simulink model "debugECDD"  (Simulink 7.2)
settings: Solver=ode1  StartTime=0.0  StopTime=50  FixedStep=0.002  RelTol=1e-3
values from neighbouring files (symbols this model uses):
  a = param.a    [DSC_Control_Analysis.m]    (also in DSC_Control_Analysis_Exp.m; DSC_Speed_Control_Analysis.m; EmpiricalTireCurves.m = 1.35; FFW_Fx.m = sqrt(curvature/(2*clothoidLength)))
  b = 1.15    [EmpiricalTireCurves.m]
  Cfls = Cfl    [EC_params_nissan.m]
  Crls = Crl    [EC_params_nissan.m]
  Iz = param.Iz    [DSC_Control_Analysis.m]    (also in DSC_Control_Analysis_Exp.m; DSC_Speed_Control_Analysis.m; EmpiricalTireCurves.m = 1300)
  K = 10    [EC_params_nissan.m]
  Ks = -10    [EC_params_nissan.m]
  Ksl = -10    [EC_params_nissan.m]
  Kt = 40000    [EC_params_nissan.m]
  Ku = -40000    [EC_params_nissan.m]
  m = 1724    [EmpiricalTireCurves.m]
  mu_s = mu_p    (= 0.6)    [EC_params_nissan.m]    (also in EmpiricalTireCurves.m = 0.55)
  Ns = 10    [EC_params_nissan.m]
  q = 1    [EC_params_nissan.m]
undefined symbols (not defined in the file or in its folder): c, Cfl, Crl, dden, denafilt, dnum, filtera, filterb, h_roll, Ifalphaparam, numafilt, param, rfl, rfr, rrl, rrr, sglu, slimFxl, slimFxu, sliml, slimMll, slimMlr, slimMul, slimMur, slimu, steering_limit, tw_m, wc
libraries: simulink x15, xpclib x3, UserBlocks x1
(part 1 of 3)
settings Model: Creator=joe4016  LastModifiedBy=joe4016
settings DataIOCC: LimitDataPoints=off

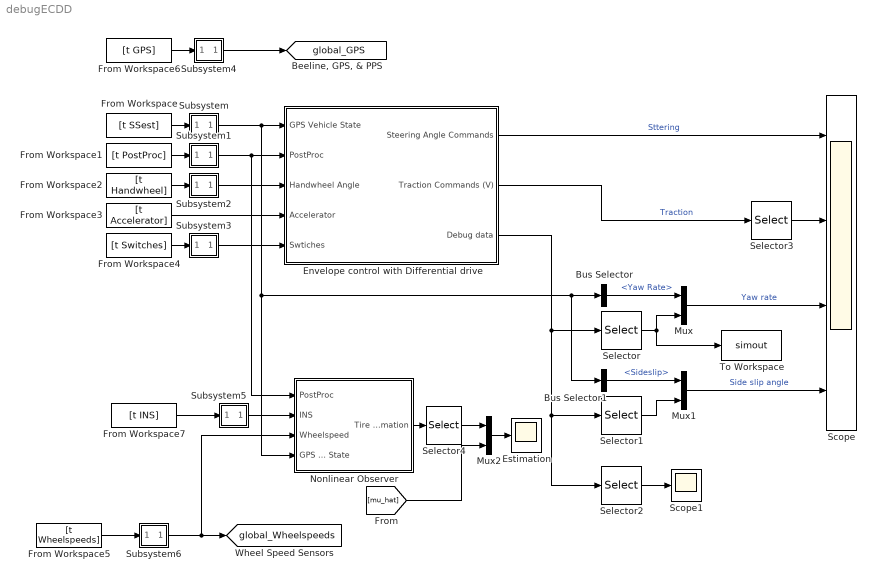
== system debugECDD ==
  Bus Selector : BusSelector  OutputSignals=Yaw Rate
  Bus Selector1 : BusSelector  OutputSignals=Sideslip
  Envelope control with Differential drive : Subsystem  AncestorBlock=UserBlocks/Envelope control with Differential drive
      mask init:
      | % get P1 parameters
      | p1_params;
      | 
      | % get params to filter handwheel angle
      | SteeringController;
      | 
      | Ts=0.002;
  Estimation : Scope
      settings: SaveName=ScopeData9
  From Workspace : FromWorkspace  VariableName=[t SSest]  SampleTime=0.002
  From Workspace1 : FromWorkspace  VariableName=[t PostProc]  SampleTime=0.002
  From Workspace2 : FromWorkspace  VariableName=[t Handwheel]  SampleTime=0.002
  From Workspace3 : FromWorkspace  VariableName=[t Accelerator]  SampleTime=0.002
  From Workspace4 : FromWorkspace  VariableName=[t Switches]  SampleTime=0.002
  From Workspace5 : FromWorkspace  VariableName=[t Wheelspeeds]  SampleTime=0.002
  From Workspace6 : FromWorkspace  VariableName=[t GPS]  SampleTime=0.002
  From Workspace7 : FromWorkspace  VariableName=[t INS]  SampleTime=0.002
  Mux : Mux  Inputs=2
  Mux1 : Mux  Inputs=2
  Mux2 : Mux  Inputs=2
  Nonlinear Observer : Subsystem
      mask init:
      | p1_params
      | nissan_steer_lookup_data
      | If_alpha_params
      | [filterb,filtera]=butter(5,0.02);
      | Ts=0.002;
      | 
      | % dryasphalt = 1;
      | % gravel = 2;
      | % 
      | % AtShoreline = [gcs '/Nonlinear Observer' '/Enable Shoreline Gravel'];
      | % 
      | % % default is dryasphalt
      | % set_param(AtShoreline, 'value', '0');
      | % 
      | % % if gravel selected, make constant AtShoreline = 1
      | % if (roadsurface == gravel)
      | %     set_param(AtShoreline, 'value', '1');
      | % end
      | %
  Scope : Scope  NumInputPorts=4
      settings: TimeRange=120  YMin=-0.4~0.5~-1.334911242603574~-0.5153846153846171  YMax=0.6~3~1.597633136094648~0.638461538461538
  Scope1 : Scope
  Selector : Selector  InputPortWidth=32  IndexOptions=Index vector (dialog)  Indices=[25 20 21]  OutputSizes=1
  Selector1 : Selector  InputPortWidth=32  IndexOptions=Index vector (dialog)  Indices=[24 22 23]  OutputSizes=1
  Selector2 : Selector  InputPortWidth=32  IndexOptions=Index vector (dialog)  Indices=16  OutputSizes=1
  Selector3 : Selector  InputPortWidth=2  IndexOptions=Index vector (dialog)  Indices=[2 1]  OutputSizes=1
  Selector4 : Selector  InputPortWidth=3  IndexOptions=Index vector (dialog)  Indices=2  OutputSizes=1
  Subsystem : Subsystem
  Subsystem1 : Subsystem
  Subsystem2 : Subsystem
  Subsystem3 : Subsystem
  Subsystem4 : Subsystem
  Subsystem5 : Subsystem
  Subsystem6 : Subsystem
  To Workspace : ToWorkspace  VariableName=simout  SampleTime=-1  SaveFormat=Array
  tag scope: global_GPS=global, global_Wheelspeeds=global
  wires:
  From Workspace/1 -> Subsystem/1(In1)
  From Workspace1/1 -> Subsystem1/1(In1)
  From Workspace2/1 -> Subsystem2/1(In1)
  From Workspace3/1 -> Envelope control with Differential drive/4(Accelerator)
  From Workspace4/1 -> Subsystem3/1(In1)
  Subsystem/1(Out1) -> Envelope control with Differential drive/1(GPS Vehicle State), Bus Selector/1, Bus Selector1/1, Nonlinear Observer/4(GPS Vehicle State)
  Subsystem1/1(Out1) -> Envelope control with Differential drive/2(PostProc), Nonlinear Observer/1(PostProc)
  Subsystem2/1(Out1) -> Envelope control with Differential drive/3(Handwheel Angle)
  Subsystem3/1(Out1) -> Envelope control with Differential drive/5(Swtiches)
  From Workspace5/1 -> Subsystem6/1(In1)
  From Workspace6/1 -> Subsystem4/1(In1)
  Subsystem4/1(Out1) -> [global_GPS]
  Envelope control with Differential drive/1(Steering Angle Commands) -> Scope/1  "Sttering"
  Envelope control with Differential drive/2(Traction Commands (V)) -> Selector3/1  "Traction"
  Envelope control with Differential drive/3(Debug data) -> Selector/1, Selector1/1, Selector2/1
  Mux/1 -> Scope/3  "Yaw rate"
  Selector/1 -> Mux/2, To Workspace/1
  Bus Selector/1 -> Mux/1  "<Yaw Rate>"
  Selector1/1 -> Mux1/2
  Bus Selector1/1 -> Mux1/1  "<Sideslip>"
  Mux1/1 -> Scope/4  "Side slip angle"
  Selector2/1 -> Scope1/1
  Selector3/1 -> Scope/2
  Subsystem5/1(Out1) -> Nonlinear Observer/2(INS)
  From Workspace7/1 -> Subsystem5/1(In1)
  Subsystem6/1(Out1) -> [global_Wheelspeeds], Nonlinear Observer/3(Wheelspeed)
  Nonlinear Observer/1(Tire Estimation) -> Selector4/1
  Mux2/1 -> Estimation/1
  [mu_hat] -> Mux2/2
  Selector4/1 -> Mux2/1

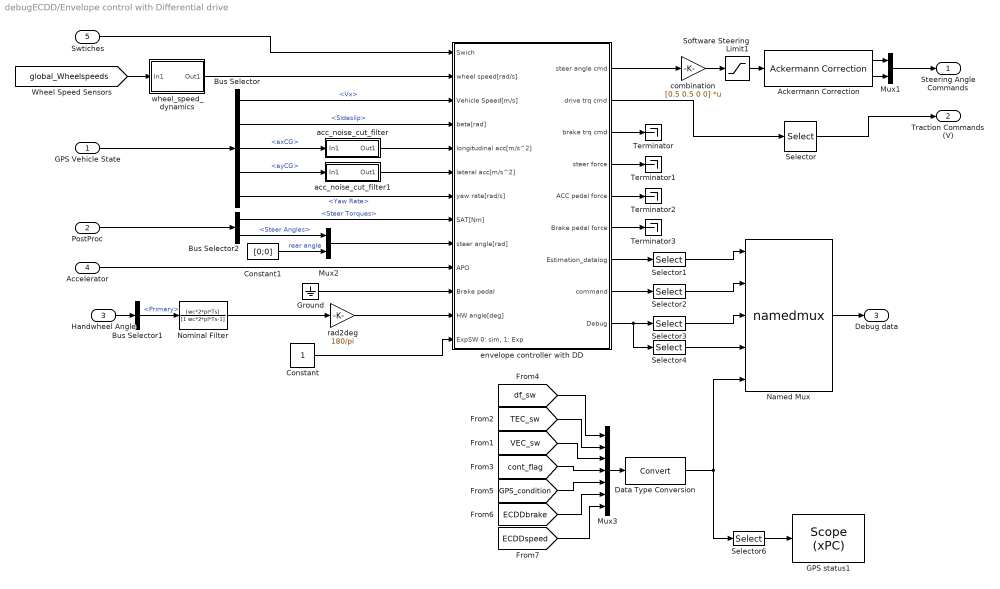
== system debugECDD/Envelope control with Differential drive ==
  GPS Vehicle State : Inport  OutDataType=sfix(16)  OutScaling=2^0
  PostProc : Inport  Port=2  OutDataType=sfix(16)  OutScaling=2^0
  Handwheel Angle : Inport  Port=3  OutDataType=sfix(16)  OutScaling=2^0
  Accelerator : Inport  Port=4  OutDataType=sfix(16)  OutScaling=2^0
  Swtiches : Inport  Port=5  OutDataType=sfix(16)  OutScaling=2^0
  Ackermann Correction : UserBlocks/Steering Controller/Ackermann Correction  SystemSampleTime=-1
  Bus Selector : BusSelector  OutputSignals=Vx,Sideslip,axCG,ayCG,Yaw Rate
  Bus Selector1 : BusSelector  OutputSignals=Primary
  Bus Selector2 : BusSelector  OutputSignals=Steer Torques,Steer Angles
  Constant : Constant  OutDataType=sfix(16)  OutScaling=2^0
  Constant1 : Constant  Value=[0;0]  OutDataType=sfix(16)  OutScaling=2^0
  Data Type Conversion : DataTypeConversion  OutDataType=sfix(16)  OutScaling=2^0
  GPS status1 : xpclib/Misc./Scope (xPC)   SystemSampleTime=-1  scopeno=2  scopetype=Target  autostart=on  viewmode=Numerical  formatstr='%15.6f'  grid=on  ylimits=[-10,10]  nosamples=round(1/Ts)  noprepostsamples=0  interleave=1  triggermode=FreeRun  triggersignal=1  triggerlevel=0.0  triggerslope=Either  triggerscope=1  triggersample=0  filename=data.dat  mode=Lazy  writesize=512  autorestart=off
  Ground : Ground
  Mux1 : Mux  Inputs=2
  Mux2 : Mux  Inputs=2
  Mux3 : Mux  Inputs=7
  Named Mux : S-Function  FunctionName=namedmux  Parameters=inputcount,inputsizes  EnableBusSupport=off  mask{fname=datadescTCS}
      mask prompts: fname "Data description function name"
      mask help:
      | Combines input signals into a single output vector, according to a structure that provides the names and sizes of each signal.
      |
      | The parameter below should be set to the name of a function which returns a 1xN structure array, where N is the number of input signals.  The structure should contain fields "size" which specifies the width of the input signal, and "name" which specifies its name.
      mask init:
      | desc=eval(fname);
      | %if(class(desc)~='cell')
      | %	error('Incorrect description');
      | %end
      | inputcount=length(desc);
      | if((inputcount<1)|(inputcount>50))
      | 	error('Inappropriate number of inputs.');
      | end
      | 
      | inputsizes=[desc.size];
      | 
      | x=min(inputcount*ones(1,50),1:50);
      mask Display:
      | port_label('input',x(1),desc(x(1)).name);
      | port_label('input',x(2),desc(x(2)).name);
      | port_label('input',x(3),desc(x(3)).name);
      | port_label('input',x(4),desc(x(4)).name);
      | port_label('input',x(5),desc(x(5)).name);
      | port_label('input',x(6),desc(x(6)).name);
      | port_label('input',x(7),desc(x(7)).name);
      | port_label('input',x(8),desc(x(8)).name);
      | port_label('input',x(9),desc(x(9)).name);
      | port_label('input',x(10),desc(x(10)).name);
      | port_label('input',x(11),desc(x(11)).name);
      | port_label('input',x(12),desc(x(12)).name);
      | port_label('input',x(13),desc(x(13)).name);
      | port_label('input',x(14),desc(x(14)).name);
      | port_label('input',x(15),desc(x(15)).name);
      | port_label('input',x(16),desc(x(16)).name);
      | port_label('input',x(17),desc(x(17)).name);
      | port_label('input',x(18),desc(x(18)).name);
      | port_label('input',x(19),desc(x(19)).name);
      | port_label('input',x(20),desc(x(20)).name);
      | port_label('input',x(21),desc(x(21)).name);
      | port_label('input',x(22),desc(x(22)).name);
      | port_label('input',x(23),desc(x(23)).name);
      | port_label('input',x(24),desc(x(24)).name);
      | port_label('input',x(25),desc(x(25)).name);
      | port_label('input',x(26),desc(x(26)).name);
      | port_label('input',x(27),desc(x(27)).name);
      | port_label('input',x(28),desc(x(28)).name);
      | port_label('input',x(29),desc(x(29)).name);
      | port_label('input',x(30),desc(x(30)).name);
  Nominal Filter : DiscreteFilter  Numerator=[wc*2*pi*Ts]  Denominator=[1 wc*2*pi*Ts-1]  SampleTime=Ts
  Selector : Selector  InputPortWidth=4  IndexOptions=Index vector (dialog)  Indices=[4 3]  OutputSizes=1
  Selector1 : Selector  InputPortWidth=17  IndexOptions=Index vector (dialog)  Indices=[1:4]  OutputSizes=1
  Selector2 : Selector  InputPortWidth=9  IndexOptions=Index vector (dialog)  Indices=[7:9]  OutputSizes=1
  Selector3 : Selector  InputPortWidth=19  IndexOptions=Index vector (dialog)  Indices=[1:8]  OutputSizes=1
  Selector4 : Selector  InputPortWidth=19  IndexOptions=Index vector (dialog)  Indices=[9,11:19]  OutputSizes=1
  Selector6 : Selector  InputPortWidth=7  IndexOptions=Index vector (dialog)  Indices=[4:7]  OutputSizes=1
  Software Steering Limit1 : Saturate  UpperLimit=steering_limit*pi/180  LowerLimit=-steering_limit*pi/180
  Terminator{,1..3} (4 alike) : Terminator
  acc_noise_cut_filter : Subsystem
      mask init:
      | [numafilt,denafilt]=butter(2,0.02);
  acc_noise_cut_filter1 : Subsystem
      mask init:
      | [numafilt,denafilt]=butter(2,0.02);
  combination : Gain  Gain=[0.5 0.5 0 0]  Multiplication=Matrix(K*u)  ParameterDataType=sfix(16)  ParameterScaling=2^0  OutDataType=sfix(16)  OutScaling=2^0
  envelope controller with DD : Subsystem
      mask init:
      | p1_params
  rad2deg : Gain  Gain=180/pi  ParameterDataType=sfix(16)  ParameterScaling=2^0  OutDataType=sfix(16)  OutScaling=2^0
  wheel_speed_dynamics : Subsystem
      mask init:
      | p1_params
      | EC_params_nissan
      | [filterb,filtera]=butter(2,0.03);
  Steering Angle Commands : Outport  OutDataType=sfix(16)  OutScaling=2^0
  Traction Commands (V) : Outport  Port=2  OutDataType=sfix(16)  OutScaling=2^0
  Debug data : Outport  Port=3  OutDataType=sfix(16)  OutScaling=2^0
  wires:
  Mux3/1 -> Data Type Conversion/1
  Swtiches/1 -> envelope controller with DD/1(Swich)
  envelope controller with DD/1(steer angle cmd) -> combination/1
  [global_Wheelspeeds] -> wheel_speed_dynamics/1(In1)
  wheel_speed_dynamics/1(Out1) -> envelope controller with DD/2(wheel speed[rad/s])
  Bus Selector/4 -> acc_noise_cut_filter1/1(In1)  "<ayCG>"
  Bus Selector/3 -> acc_noise_cut_filter/1(In1)  "<axCG>"
  Bus Selector/2 -> envelope controller with DD/4(beta[rad])  "<Sideslip>"
  Bus Selector/5 -> envelope controller with DD/7(yaw rate[rad/s])  "<Yaw Rate>"
  Bus Selector/1 -> envelope controller with DD/3(Vehicle Speed[m/s])  "<Vx>"
  Accelerator/1 -> envelope controller with DD/10(APO)
  Constant1/1 -> Mux2/2  "rear angle"
  Bus Selector2/2 -> Mux2/1  "<Steer Angles>"
  Bus Selector2/1 -> envelope controller with DD/8(SAT[Nm])  "<Steer Torques>"
  PostProc/1 -> Bus Selector2/1
  GPS Vehicle State/1 -> Bus Selector/1
  Constant/1 -> envelope controller with DD/13("ExpSW 0: sim, 1: Exp")
  rad2deg/1 -> envelope controller with DD/12(HW angle[deg])
  Nominal Filter/1 -> rad2deg/1
  Bus Selector1/1 -> Nominal Filter/1  "<Primary>"
  Named Mux/1 -> Debug data/1
  Selector3/1 -> Named Mux/3
  Selector2/1 -> Named Mux/2
  Selector1/1 -> Named Mux/1
  envelope controller with DD/9(Debug) -> Selector4/1, Selector3/1
  envelope controller with DD/8(command) -> Selector2/1
  envelope controller with DD/2(drive trq cmd) -> Selector/1
  envelope controller with DD/7(Estimation_datalog) -> Selector1/1
  envelope controller with DD/6(Brake pedal force) -> Terminator3/1
  envelope controller with DD/5(ACC pedal force) -> Terminator2/1
  envelope controller with DD/4(steer force) -> Terminator1/1
  envelope controller with DD/3(brake trq cmd) -> Terminator/1
  Selector/1 -> Traction Commands (V)/1
  combination/1 -> Software Steering Limit1/1
  Mux1/1 -> Steering Angle Commands/1
  Ackermann Correction/2 -> Mux1/2
  Ackermann Correction/1 -> Mux1/1
  Software Steering Limit1/1 -> Ackermann Correction/1
  Mux2/1 -> envelope controller with DD/9(steer angle[rad])
  Ground/1 -> envelope controller with DD/11(Brake pedal)
  Handwheel Angle/1 -> Bus Selector1/1
  Data Type Conversion/1 -> Selector6/1, Named Mux/5
  acc_noise_cut_filter/1(Out1) -> envelope controller with DD/5(longitudinal acc[m/s^2])
  acc_noise_cut_filter1/1(Out1) -> envelope controller with DD/6(lateral acc[m/s^2])
  Selector4/1 -> Named Mux/4
  [df_sw] -> Mux3/1
  [TEC_sw] -> Mux3/2
  [VEC_sw] -> Mux3/3
  [cont_flag] -> Mux3/4
  [GPS_condition] -> Mux3/5
  [ECDDbrake] -> Mux3/6
  [ECDDspeed] -> Mux3/7
  Selector6/1 -> GPS status1/1

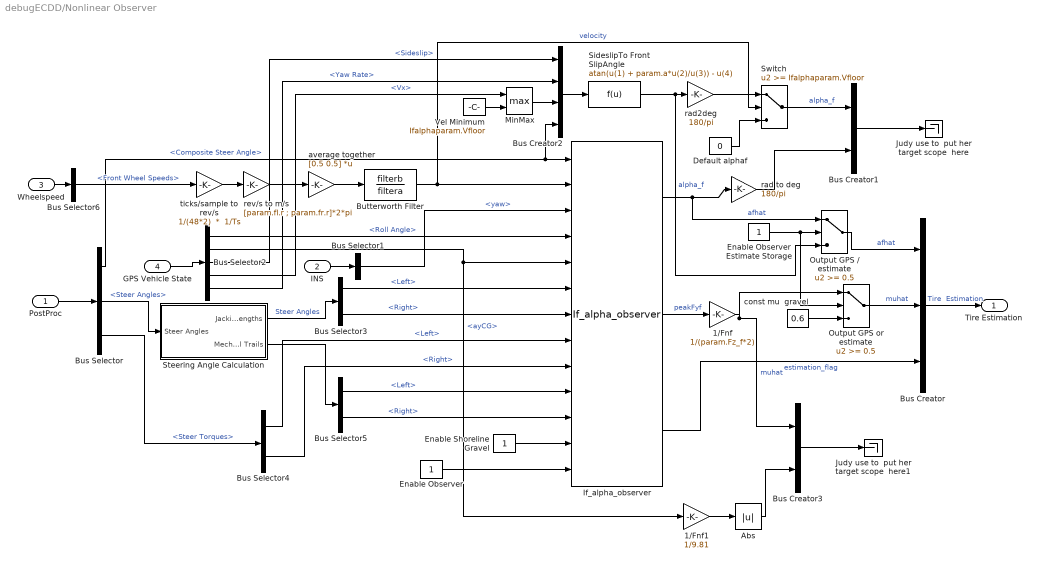
== system debugECDD/Nonlinear Observer ==
  PostProc : Inport  OutDataType=sfix(16)  OutScaling=2^0
  INS : Inport  Port=2  OutDataType=sfix(16)  OutScaling=2^0
  Wheelspeed : Inport  Port=3  OutDataType=sfix(16)  OutScaling=2^0
  GPS Vehicle State : Inport  Port=4  OutDataType=sfix(16)  OutScaling=2^0
  1/Fnf : Gain  Gain=1/(param.Fz_f*2)  ParameterDataType=sfix(16)  ParameterScaling=2^0  OutDataType=sfix(16)  OutScaling=2^0
  1/Fnf1 : Gain  Gain=1/9.81  ParameterDataType=sfix(16)  ParameterScaling=2^0  OutDataType=sfix(16)  OutScaling=2^0
  Abs : Abs
  Bus Creator : BusCreator  Inputs=3
  Bus Creator1 : BusCreator  Inputs=2
  Bus Creator2 : BusCreator
  Bus Creator3 : BusCreator  Inputs=2
  Bus Selector : BusSelector  OutputSignals=Composite Steer Angle,Steer Angles,Steer Torques
  Bus Selector1 : BusSelector  OutputSignals=yaw
  Bus Selector2 : BusSelector  OutputSignals=Roll Angle,ayCG,Sideslip,Vx,Yaw Rate
  Bus Selector3 : BusSelector  OutputSignals=Left,Right
  Bus Selector4 : BusSelector  OutputSignals=Left,Right
  Bus Selector5 : BusSelector  OutputSignals=Left,Right
  Bus Selector6 : BusSelector  OutputSignals=Front Wheel Speeds
  Butterworth Filter : DiscreteFilter  Numerator=filterb  Denominator=filtera  SampleTime=Ts
  Default alphaf : Constant  Value=0  OutDataType=sfix(16)  OutScaling=2^0
  Enable Observer : Constant  OutDataType=sfix(16)  OutScaling=2^0
  Enable Shoreline Gravel : Constant  OutDataType=sfix(16)  OutScaling=2^0
  Enable Observer Estimate Storage : Constant  OutDataType=sfix(16)  OutScaling=2^0
  If_alpha_observer : S-Function  FunctionName=If_alpha_observer  Parameters=|  EnableBusSupport=off
      | Ifalphaparam.tp_window, Ifalphaparam.FIRwindow, Ifalphaparam.IFwindow, param.Fz_f, Ifalphaparam.mu_peak_nom, param.fl.fw, param.fl.Jw, param.fl.bw,
      | 
      | 
      | 
      | 
      | 
      | 
      | 
      | 
      | param.fr.fw, param.fr.Jw, param.fr.bw, param.a, param.b, param.m, Ifalphaparam.hf, param.tw, param.Iz, Ifalphaparam.Kaf0, Ts, Ifalphaparam.phiceil,
      | 
      | 
      | 
      | 
      | 
      | 
      | 
      | 
      | Ifalphaparam.Vfloor, Ifalphaparam.ayfloor, Ifalphaparam.tp0, Ifalphaparam.Caf, Ifalphaparam.Car, Ifalphaparam.Caf_shoreline_sf, Ifalphaparam.mu_slip_nom, 
      | 
      | 
      | 
      | 
      | 
      | 
      | 
      | 
      | Ifalphaparam.alpha_thres, Ifalphaparam.tpthres_sf, Ifalphaparam.Kphif, Ifalphaparam.afhatceil, Ifalphaparam.Kaf_sf_Shoreline, Ifalphaparam.Kaf_sf_asphalt,
      | 
      | 
      | 
      | 
      | 
      | 
      | 
      | 
      | Ifalphaparam.Car_shoreline_sf, Ifalphaparam.alphafoffset, Ifalphaparam.alpharoffset
  Judy use to  put her target scope  here : Terminator
  Judy use to  put her target scope  here1 : Terminator
  MinMax : MinMax  Function=max  Inputs=2  OutDataType=sfix(16)  OutScaling=2^0
  Output GPS / estimate : Switch  Threshold=0.5
  Output GPS or estimate : Switch  Threshold=0.5
  SideslipTo Front SlipAngle : Fcn  Expr=atan(u(1) + param.a*u(2)/u(3)) - u(4)
  Steering Angle Calculation : Subsystem
      mask init:
      | p1_params
      | nissan_steer_lookup_data
  Switch : Switch  Threshold=Ifalphaparam.Vfloor
  Vel Minimum : Constant  Value=Ifalphaparam.Vfloor  OutDataType=sfix(16)  OutScaling=2^0
  average together : Gain  Gain=[0.5 0.5]  Multiplication=Matrix(K*u)  ParameterDataType=sfix(16)  ParameterScaling=2^0  OutDataType=sfix(16)  OutScaling=2^0
  const mu  gravel : Constant  Value=0.6  OutDataType=sfix(16)  OutScaling=2^0
  rad to deg : Gain  Gain=180/pi  ParameterDataType=sfix(16)  ParameterScaling=2^0  OutDataType=sfix(16)  OutScaling=2^0
  rad2deg : Gain  Gain=180/pi  ParameterDataType=sfix(16)  ParameterScaling=2^0  OutDataType=sfix(16)  OutScaling=2^0
  rev/s to m/s : Gain  Gain=[param.fl.r ; param.fr.r]*2*pi  ParameterDataType=sfix(16)  ParameterScaling=2^0  OutDataType=sfix(16)  OutScaling=2^0
  ticks/sample to rev/s : Gain  Gain="1/(48*2)  *  1/Ts"  ParameterDataType=sfix(16)  ParameterScaling=2^0  OutDataType=sfix(16)  OutScaling=2^0
  Tire Estimation : Outport  OutDataType=sfix(16)  OutScaling=2^0
  wires:
  PostProc/1 -> Bus Selector/1
  Bus Creator/1 -> Tire Estimation/1  "Tire  Estimation"
  INS/1 -> Bus Selector1/1
  GPS Vehicle State/1 -> Bus Selector2/1
  Wheelspeed/1 -> Bus Selector6/1
  ticks/sample to rev/s/1 -> rev/s to m/s/1
  rev/s to m/s/1 -> average together/1
  average together/1 -> Butterworth Filter/1
  Bus Selector/2 -> Steering Angle Calculation/1(Steer Angles)  "<Steer Angles>"
  Bus Selector/1 -> If_alpha_observer/1, Bus Creator2/4  "<Composite Steer Angle>"
  Butterworth Filter/1 -> If_alpha_observer/2, Switch/2  "velocity"
  Bus Selector1/1 -> If_alpha_observer/3  "<yaw>"
  Bus Selector2/1 -> If_alpha_observer/4  "<Roll Angle>"
  Bus Selector2/2 -> If_alpha_observer/5, 1/Fnf1/1  "<ayCG>"
  Steering Angle Calculation/1(Jacking Arm Lengths) -> Bus Selector3/1  "Steer Angles"
  Bus Selector3/1 -> If_alpha_observer/6  "<Left>"
  Bus Selector3/2 -> If_alpha_observer/7  "<Right>"
  Bus Selector/3 -> Bus Selector4/1  "<Steer Torques>"
  Bus Selector4/1 -> If_alpha_observer/8  "<Left>"
  Bus Selector4/2 -> If_alpha_observer/9  "<Right>"
  Steering Angle Calculation/2(Mechanical Trails) -> Bus Selector5/1
  Bus Selector5/1 -> If_alpha_observer/10  "<Left>"
  Bus Selector5/2 -> If_alpha_observer/11  "<Right>"
  If_alpha_observer/1 -> rad to deg/1, Output GPS / estimate/1  "afhat"
  If_alpha_observer/3 -> Bus Creator/3  "estimation_flag"
  Bus Selector2/3 -> Bus Creator2/1  "<Sideslip>"
  Bus Creator2/1 -> SideslipTo Front SlipAngle/1
  SideslipTo Front SlipAngle/1 -> rad2deg/1, Output GPS / estimate/3  "alpha_f"
  If_alpha_observer/2 -> 1/Fnf/1  "peakFyf"
  Enable Shoreline Gravel/1 -> If_alpha_observer/12
  1/Fnf1/1 -> Abs/1
  Bus Creator3/1 -> Judy use to  put her target scope  here1/1
  Abs/1 -> Bus Creator3/2
  rad to deg/1 -> Bus Creator1/2
  Bus Creator1/1 -> Judy use to  put her target scope  here/1
  MinMax/1 -> Bus Creator2/3
  Vel Minimum/1 -> MinMax/2
  rad2deg/1 -> Switch/1
  Switch/1 -> Bus Creator1/1  "alpha_f"
  1/Fnf/1 -> Bus Creator3/1, Output GPS or estimate/1  "muhat"
  Default alphaf/1 -> Switch/3
  Enable Observer Estimate Storage/1 -> Output GPS / estimate/2, Output GPS or estimate/2
  Output GPS / estimate/1 -> Bus Creator/1  "afhat"
  Output GPS or estimate/1 -> Bus Creator/2  "muhat"
  const mu  gravel/1 -> Output GPS or estimate/3
  Bus Selector2/4 -> MinMax/1  "<Vx>"
  Bus Selector2/5 -> Bus Creator2/2  "<Yaw Rate>"
  Enable Observer/1 -> If_alpha_observer/13
  Bus Selector6/1 -> ticks/sample to rev/s/1  "<Front Wheel Speeds>"

== system debugECDD/Subsystem ==
  In1 : Inport  OutDataType=sfix(16)  OutScaling=2^0
  Demux : Demux  Outputs=21
  Mux : Mux  Inputs=21
  Out1 : Outport  OutDataType=sfix(16)  OutScaling=2^0
  wires:
  In1/1 -> Demux/1
  Mux/1 -> Out1/1
  Demux/1 -> Mux/1  "Yaw Angle"
  Demux/2 -> Mux/2  "Yaw Gyro Sf"
  Demux/3 -> Mux/3  "Yaw Gyro Bias"
  Demux/4 -> Mux/4  "Yaw Rate"
  Demux/5 -> Mux/5  "Roll Angle"
  Demux/6 -> Mux/6  "Roll Gyro Sf"
  Demux/7 -> Mux/7  "Roll Gyro Bias"
  Demux/8 -> Mux/8  "Roll Rate"
  Demux/9 -> Mux/9  "Vx"
  Demux/10 -> Mux/10  "ax bias"
  Demux/11 -> Mux/11  "axCG"
  Demux/12 -> Mux/12  "VyCG"
  Demux/13 -> Mux/13  "ay bias"
  Demux/14 -> Mux/14  "ayCG"
  Demux/15 -> Mux/15  "Sideslip"
  Demux/16 -> Mux/16  "Pos E"
  Demux/17 -> Mux/17  "Pos N"
  Demux/18 -> Mux/18  "OEM4 Delay"
  Demux/19 -> Mux/19  "Beeline Delay"
  Demux/20 -> Mux/20  "OEM4 Update"
  Demux/21 -> Mux/21  "Beeline Update"

== system debugECDD/Subsystem1 ==
  In1 : Inport  OutDataType=sfix(16)  OutScaling=2^0
  Bus Creator : BusCreator  Inputs=3
  Bus Creator1 : BusCreator  Inputs=2
  Bus Creator2 : BusCreator  Inputs=2
  Demux : Demux  Outputs=5
  Out1 : Outport  OutDataType=sfix(16)  OutScaling=2^0
  wires:
  Bus Creator/1 -> Out1/1
  In1/1 -> Demux/1
  Demux/3 -> Bus Creator/2  "Composite Steer Angle"
  Bus Creator2/1 -> Bus Creator/3  "Steer Torques"
  Bus Creator1/1 -> Bus Creator/1  "Steer Angles"
  Demux/1 -> Bus Creator1/1  "Left"
  Demux/2 -> Bus Creator1/2  "Right"
  Demux/5 -> Bus Creator2/2  "Right"
  Demux/4 -> Bus Creator2/1  "Left"

== system debugECDD/Subsystem2 ==
  In1 : Inport  OutDataType=sfix(16)  OutScaling=2^0
  Demux : Demux  Outputs=3
  Mux : Mux  Inputs=3
  Out1 : Outport  OutDataType=sfix(16)  OutScaling=2^0
  wires:
  Mux/1 -> Out1/1
  In1/1 -> Demux/1
  Demux/1 -> Mux/1  "Primary"
  Demux/2 -> Mux/2  "Secondary"
  Demux/3 -> Mux/3  "Encoder Fault Status"

== system debugECDD/Subsystem3 ==
  In1 : Inport  OutDataType=sfix(16)  OutScaling=2^0
  Constant : Constant  OutDataType=sfix(16)  OutScaling=2^0
  Constant1 : Constant  OutDataType=sfix(16)  OutScaling=2^0
  Demux : Demux
  Manual Switch : simulink/Signal Routing/Manual Switch  SystemSampleTime=-1  sw=1  action=0  varsize=off
  Manual Switch1 : simulink/Signal Routing/Manual Switch  SystemSampleTime=-1  sw=1  action=0  varsize=off
  Mux : Mux
  Out1 : Outport  OutDataType=sfix(16)  OutScaling=2^0
  wires:
  In1/1 -> Demux/1
  Mux/1 -> Out1/1
  Manual Switch/1 -> Mux/1  "Fault Switch"
  Manual Switch1/1 -> Mux/2  "Auto-Steer Switch"
  Demux/3 -> Mux/3  "Cruise Control Switch"
  Demux/4 -> Mux/4  "Brake Pedal Signal"
  Demux/2 -> Manual Switch1/2  "Auto-Steer Switch"
  Demux/1 -> Manual Switch/2  "Fault Switch"
  Constant/1 -> Manual Switch/1
  Constant1/1 -> Manual Switch1/1

== system debugECDD/Subsystem4 ==
  In1 : Inport  OutDataType=sfix(16)  OutScaling=2^0
  Demux : Demux  Outputs=[10 6 1 6 2]
  Demux1 : Demux  Outputs=6
  Demux2 : Demux  Outputs=10
  Mux : Mux  Inputs=5
  Mux1 : Mux  Inputs=6
  Mux2 : Mux  Inputs=10
  Out1 : Outport  OutDataType=sfix(16)  OutScaling=2^0
  wires:
  In1/1 -> Demux/1
  Mux/1 -> Out1/1
  Demux/2 -> Demux1/1
  Demux1/1 -> Mux1/1
  Demux1/2 -> Mux1/2
  Demux1/3 -> Mux1/3
  Demux1/4 -> Mux1/4
  Demux1/5 -> Mux1/5
  Demux1/6 -> Mux1/6  "Velocity Solution Status"
  Demux/1 -> Demux2/1
  Demux/3 -> Mux/3
  Demux/4 -> Mux/4
  Demux/5 -> Mux/5
  Demux2/1 -> Mux2/1
  Demux2/2 -> Mux2/2
  Demux2/3 -> Mux2/3
  Demux2/4 -> Mux2/4  "Attitude Status"
  Demux2/5 -> Mux2/5
  Demux2/6 -> Mux2/6
  Demux2/7 -> Mux2/7
  Demux2/8 -> Mux2/8
  Demux2/9 -> Mux2/9
  Demux2/10 -> Mux2/10
  Mux2/1 -> Mux/1
  Mux1/1 -> Mux/2

== system debugECDD/Subsystem5 ==
  In1 : Inport  OutDataType=sfix(16)  OutScaling=2^0
  Bus Creator : BusCreator  Inputs=6
  Demux : Demux  Outputs=6
  Out1 : Outport  OutDataType=sfix(16)  OutScaling=2^0
  wires:
  In1/1 -> Demux/1
  Demux/2 -> Bus Creator/2  "ax"
  Demux/3 -> Bus Creator/3  "roll"
  Demux/4 -> Bus Creator/4  "ay"
  Demux/5 -> Bus Creator/5  "pitch"
  Demux/6 -> Bus Creator/6  "az"
  Demux/1 -> Bus Creator/1  "yaw"
  Bus Creator/1 -> Out1/1

== system debugECDD/Subsystem6 ==
  In1 : Inport  OutDataType=sfix(16)  OutScaling=2^0
  Bus Creator6 : BusCreator  Inputs=2
  Demux : Demux  Outputs=[2 2]
  Out1 : Outport  OutDataType=sfix(16)  OutScaling=2^0
  wires:
  Bus Creator6/1 -> Out1/1
  In1/1 -> Demux/1
  Demux/1 -> Bus Creator6/1  "Front Wheel Speeds"
  Demux/2 -> Bus Creator6/2  "Rear Wheel Speeds"

== system debugECDD/Envelope control with Differential drive/acc_noise_cut_filter ==
  In1 : Inport  OutDataType=sfix(16)  OutScaling=2^0
  Butterworth Filter : DiscreteFilter  Numerator=numafilt  Denominator=denafilt  SampleTime=0.002
  Out1 : Outport  OutDataType=sfix(16)  OutScaling=2^0
  wires:
  Butterworth Filter/1 -> Out1/1
  In1/1 -> Butterworth Filter/1

== system debugECDD/Envelope control with Differential drive/acc_noise_cut_filter1 ==
  In1 : Inport  OutDataType=sfix(16)  OutScaling=2^0
  Butterworth Filter : DiscreteFilter  Numerator=numafilt  Denominator=denafilt  SampleTime=0.002
  Out1 : Outport  OutDataType=sfix(16)  OutScaling=2^0
  wires:
  In1/1 -> Butterworth Filter/1
  Butterworth Filter/1 -> Out1/1

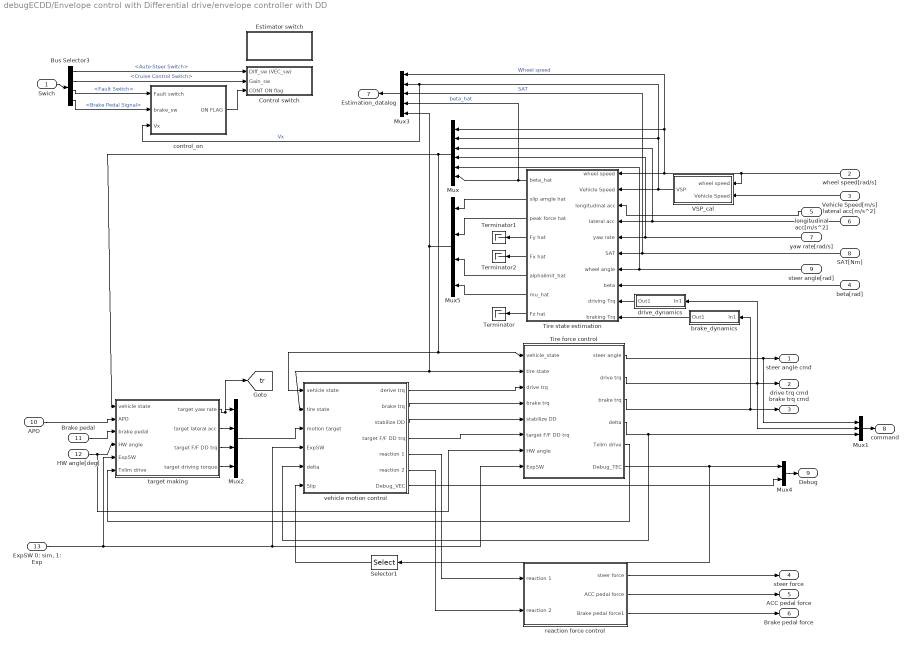
== system debugECDD/Envelope control with Differential drive/envelope controller with DD ==
  Swich : Inport  OutDataType=sfix(16)  OutScaling=2^0
  wheel speed[rad/s] : Inport  Orientation=left  Port=2  OutDataType=sfix(16)  OutScaling=2^0
  Vehicle Speed[m/s] : Inport  Orientation=left  Port=3  OutDataType=sfix(16)  OutScaling=2^0
  beta[rad] : Inport  Orientation=left  Port=4  OutDataType=sfix(16)  OutScaling=2^0
  longitudinal acc[m/s^2] : Inport  Orientation=left  Port=5  OutDataType=sfix(16)  OutScaling=2^0
  lateral acc[m/s^2] : Inport  Orientation=left  Port=6  OutDataType=sfix(16)  OutScaling=2^0
  yaw rate[rad/s] : Inport  Orientation=left  Port=7  OutDataType=sfix(16)  OutScaling=2^0
  SAT[Nm] : Inport  Orientation=left  Port=8  OutDataType=sfix(16)  OutScaling=2^0
  steer angle[rad] : Inport  Orientation=left  Port=9  OutDataType=sfix(16)  OutScaling=2^0
  APO : Inport  Port=10  OutDataType=sfix(16)  OutScaling=2^0
  Brake pedal : Inport  Port=11  OutDataType=sfix(16)  OutScaling=2^0
  HW angle[deg] : Inport  Port=12  OutDataType=sfix(16)  OutScaling=2^0
  "ExpSW 0: sim, 1: Exp" : Inport  Port=13  OutDataType=sfix(16)  OutScaling=2^0
  Bus Selector3 : BusSelector  OutputSignals=Auto-Steer Switch,Cruise Control Switch,Fault Switch,Brake Pedal Signal
  Control switch : Subsystem
  Estimator switch : Subsystem
  Mux : Mux  Orientation=left  Inputs=6
  Mux1 : Mux  Inputs=3
  Mux2 : Mux
  Mux3 : Mux  Orientation=left  Inputs=5
  Mux4 : Mux  Inputs=2
  Mux5 : Mux  Orientation=left
  Selector1 : Selector  Orientation=left  InputPortWidth=8  IndexOptions=Index vector (dialog)  Indices=[5:6]  OutputSizes=1
  Terminator : Terminator
  Terminator1 : Terminator
  Terminator2 : Terminator
  Tire force control : Subsystem
      mask init:
      | p1_params
      | EC_params_nissan
      | load slimmap
      | [filterb,filtera]=butter(2,0.03);
  Tire state estimation : Subsystem  Orientation=left
      mask init:
      | p1_params
      | EC_params_nissan
  VSP_cal : Subsystem  Orientation=left
      mask init:
      | p1_params
      | EC_params_nissan
  brake_dynamics : Subsystem  Orientation=left
  control_on : Subsystem
  drive_dynamics : Subsystem  Orientation=left
  reaction force control : Subsystem
  target making : Subsystem
      mask init:
      | p1_params
      | EC_params_nissan
      | % FFDDmodel_cal
      | [dnum,dden]=c2dm([1 0],[0.1 1],0.002,'tustin');
  vehicle motion control : Subsystem
      mask init:
      | p1_params
      | EC_params_nissan
      | load stableareamap.mat
  steer angle cmd : Outport  OutDataType=sfix(16)  OutScaling=2^0
  drive trq cmd : Outport  Port=2  OutDataType=sfix(16)  OutScaling=2^0
  brake trq cmd : Outport  Port=3  OutDataType=sfix(16)  OutScaling=2^0
  steer force : Outport  Port=4  OutDataType=sfix(16)  OutScaling=2^0
  ACC pedal force : Outport  Port=5  OutDataType=sfix(16)  OutScaling=2^0
  Brake pedal force : Outport  Port=6  OutDataType=sfix(16)  OutScaling=2^0
  Estimation_datalog : Outport  Orientation=left  Port=7  OutDataType=sfix(16)  OutScaling=2^0
  command : Outport  Port=8  OutDataType=sfix(16)  OutScaling=2^0
  Debug : Outport  Port=9  OutDataType=sfix(16)  OutScaling=2^0
  tag scope: tr=global
  wires:
  Bus Selector3/1 -> Control switch/1(Diff_sw (VEC_sw))  "<Auto-Steer Switch>"
  Bus Selector3/4 -> control_on/2(brake_sw)  "<Brake Pedal Signal>"
  Bus Selector3/3 -> control_on/1(Fault switch)  "<Fault Switch>"
  Swich/1 -> Bus Selector3/1
  control_on/1(ON FLAG) -> Control switch/3(CONT ON flag)
  longitudinal acc[m/s^2]/1 -> Tire state estimation/3(longitudinal acc)
  "ExpSW 0: sim, 1: Exp"/1 -> Tire force control/8(ExpSW), vehicle motion control/4(ExpSW), target making/5(ExpSW)
  Mux4/1 -> Debug/1
  vehicle motion control/7(Debug_VEC) -> Mux4/2
  Tire force control/6(Debug_TEC) -> Mux4/1, Selector1/1
  Tire state estimation/6(alphalimit_hat) -> Mux5/3
  Tire state estimation/7(mu_hat) -> Mux5/4
  Tire state estimation/5(Fx hat) -> Terminator2/1
  Tire state estimation/4(Fy hat) -> Terminator1/1
  Mux1/1 -> command/1
  Vehicle Speed[m/s]/1 -> VSP_cal/2(Vehicle Speed)
  VSP_cal/1(VSP) -> Tire state estimation/2(Vehicle Speed), Mux/2, Mux3/2, control_on/3(Vx)  "Vx"
  Tire state estimation/1(beta_hat) -> Mux3/4, Mux/6  "beta_hat"
  beta[rad]/1 -> Tire state estimation/8(beta)
  target making/1(target yaw rate) -> [tr], Mux2/1
  Tire force control/4(delta) -> Mux1/3, vehicle motion control/5(delta)
  steer angle[rad]/1 -> Tire state estimation/7(wheel angle), Mux/5
  brake_dynamics/1(Out1) -> Tire state estimation/10(braking Trq)
  drive_dynamics/1(Out1) -> Tire state estimation/9(driving Trq)
  Mux5/1 -> Mux3/5, Tire force control/2(tire state), vehicle motion control/2(tire state)
  Mux/1 -> target making/1(vehicle state), Tire force control/1(vehicle_state), vehicle motion control/1(vehicle state)
  vehicle motion control/3(stabilize DD) -> Tire force control/5(stabilize DD)
  Mux3/1 -> Estimation_datalog/1
  Tire state estimation/8(Fz hat) -> Terminator/1
  Tire state estimation/3(peak force hat) -> Mux5/2
  Tire state estimation/2(slip amgle hat) -> Mux5/1
  SAT[Nm]/1 -> Tire state estimation/6(SAT), Mux3/3  "SAT"
  wheel speed[rad/s]/1 -> VSP_cal/1(wheel speed), Tire state estimation/1(wheel speed), Mux3/1, Mux/1  "Wheel speed"
  reaction force control/3(Brake pedal force1) -> Brake pedal force/1
  reaction force control/2(ACC pedal force) -> ACC pedal force/1
  reaction force control/1(steer force) -> steer force/1
  vehicle motion control/6(reaction 2) -> reaction force control/2(reaction 2)
  vehicle motion control/5(reaction 1) -> reaction force control/1(reaction 1)
  vehicle motion control/2(brake trq) -> Tire force control/4("brake trq ")
  vehicle motion control/1(derive trq) -> Tire force control/3("drive trq ")
  Tire force control/3(brake trq) -> brake_dynamics/1(In1), brake trq cmd/1
  Tire force control/2(drive trq) -> Mux1/2, drive_dynamics/1(In1), drive trq cmd/1
  Tire force control/1(steer angle) -> Mux1/1, steer angle cmd/1
  Mux2/1 -> vehicle motion control/3(motion target)
  target making/3(target F/F DD trq) -> Mux2/3
  target making/2(target lateral acc) -> Mux2/2
  Brake pedal/1 -> target making/3(brake pedal)
  APO/1 -> target making/2(APO)
  HW angle[deg]/1 -> Tire force control/7(HW angle), target making/4(HW angle)
  yaw rate[rad/s]/1 -> Tire state estimation/5(yaw rate), Mux/4
  lateral acc[m/s^2]/1 -> Tire state estimation/4(lateral acc), Mux/3
  target making/4(target driving torque) -> Mux2/4
  Tire force control/5(Txlim drive) -> target making/6(Txlim drive)
  Selector1/1 -> vehicle motion control/6(Slip)
  vehicle motion control/4(target F/F DD trq) -> Tire force control/6(target F/F DD trq)
  Bus Selector3/2 -> Control switch/2(Gain_sw)  "<Cruise Control Switch>"

== system debugECDD/Envelope control with Differential drive/wheel_speed_dynamics ==
  In1 : Inport  OutDataType=sfix(16)  OutScaling=2^0
  Butterworth Filter{,1..3} (4 alike) : DiscreteFilter  Numerator=filterb  Denominator=filtera  SampleTime=0.002
  Demux : Demux
  Mux : Mux
  rev/s to rad/s : Gain  Gain=2*pi  ParameterDataType=sfix(16)  ParameterScaling=2^0  OutDataType=sfix(16)  OutScaling=2^0
  ticks/sample to rev/s : Gain  Gain="1/(48*2)  *  1/Ts"  ParameterDataType=sfix(16)  ParameterScaling=2^0  OutDataType=sfix(16)  OutScaling=2^0
  Out1 : Outport  OutDataType=sfix(16)  OutScaling=2^0
  wires:
  In1/1 -> ticks/sample to rev/s/1
  rev/s to rad/s/1 -> Demux/1
  ticks/sample to rev/s/1 -> rev/s to rad/s/1
  Butterworth Filter3/1 -> Mux/4
  Butterworth Filter2/1 -> Mux/3
  Butterworth Filter1/1 -> Mux/2
  Butterworth Filter/1 -> Mux/1
  Mux/1 -> Out1/1
  Demux/1 -> Butterworth Filter1/1
  Demux/2 -> Butterworth Filter/1
  Demux/3 -> Butterworth Filter3/1
  Demux/4 -> Butterworth Filter2/1

== system debugECDD/Nonlinear Observer/Steering Angle Calculation ==
  Steer Angles : Inport  OutDataType=sfix(16)  OutScaling=2^0
  Bus Creator : BusCreator  Inputs=2
  Bus Creator1 : BusCreator  Inputs=2
  Bus Selector1 : BusSelector  OutputSignals=Left,Right
  Left Steer Angle Look-up : Lookup  InputValues=sglu.fl.sa  Table=sglu.fl.ja  OutDataType=sfix(16)  OutScaling=2^0  SaturateOnIntegerOverflow=on
  Left Steer Angle Look-up1 : Lookup  InputValues=sglu.fl.sa  Table=sglu.fl.mt  OutDataType=sfix(16)  OutScaling=2^0  SaturateOnIntegerOverflow=on
  Right Steer Angle Look-up : Lookup  InputValues=sglu.fr.sa  Table=sglu.fr.ja  OutDataType=sfix(16)  OutScaling=2^0  SaturateOnIntegerOverflow=on
  Right Steer Angle Look-up1 : Lookup  InputValues=sglu.fr.sa  Table=sglu.fr.mt  OutDataType=sfix(16)  OutScaling=2^0  SaturateOnIntegerOverflow=on
  Jacking Arm Lengths : Outport  OutDataType=sfix(16)  OutScaling=2^0
  Mechanical Trails : Outport  Port=2  OutDataType=sfix(16)  OutScaling=2^0
  wires:
  Steer Angles/1 -> Bus Selector1/1
  Bus Creator/1 -> Jacking Arm Lengths/1
  Left Steer Angle Look-up/1 -> Bus Creator/1  "Left"
  Right Steer Angle Look-up/1 -> Bus Creator/2  "Right"
  Bus Creator1/1 -> Mechanical Trails/1
  Left Steer Angle Look-up1/1 -> Bus Creator1/1  "Left"
  Right Steer Angle Look-up1/1 -> Bus Creator1/2  "Right"
  Bus Selector1/1 -> Left Steer Angle Look-up/1, Left Steer Angle Look-up1/1  "<Left>"
  Bus Selector1/2 -> Right Steer Angle Look-up/1, Right Steer Angle Look-up1/1  "<Right>"

== system debugECDD/Envelope control with Differential drive/envelope controller with DD/Control switch ==
  Diff_sw (VEC_sw) : Inport  OutDataType=sfix(16)  OutScaling=2^0
  Gain_sw : Inport  Port=2  OutDataType=sfix(16)  OutScaling=2^0
  CONT ON flag : Inport  Port=3  OutDataType=sfix(16)  OutScaling=2^0
  Delay : Subsystem
  "Front tire slip angle limit switch 0 : OFF, 1: ON" : Constant  Value=0  OutDataType=sfix(16)  OutScaling=2^0
  Logical Operator{1..5} (5 alike) : Logic  AllPortsSameDT=off  OutDataTypeMode=boolean  OutDataTypeStr=boolean
  Manual Switch : simulink/Signal Routing/Manual Switch  SystemSampleTime=-1  sw=1  action=0  varsize=off
  "Safe area 0 : small, 1: large" : Constant  OutDataType=sfix(16)  OutScaling=2^0
  "Slip limit control switch 0: OFF , 1: ON" : Constant  Value=0  OutDataType=sfix(16)  OutScaling=2^0
  Step : Step  SampleTime=0
  "Tire envelope control switch 0: TEC OFF , 1: TEC ON" : Constant  OutDataType=sfix(16)  OutScaling=2^0
  Triggered Subsystem1 : Subsystem  TreatAsAtomicUnit=on
  Unit Delay : UnitDelay  X0=2  SampleTime=0.002
  "Vehicle envelope control switch 0: VEC OFF, 1:VEC ON" : Constant  OutDataType=sfix(16)  OutScaling=2^0
  "drive switch 0 : OFF(no driving force), 1 : ON" : Constant  OutDataType=sfix(16)  OutScaling=2^0
  tag scope: Boundary_sw=global, D_sw=global, Diff_gain=global, Diff_sw=global, TEC_sw=global, VEC_sw=global, cont_flag=global, df_sw=global, sliplimit_sw=global
  wires:
  CONT ON flag/1 -> Logical Operator3/1, Logical Operator4/1, [cont_flag], Logical Operator2/1
  "Front tire slip angle limit switch 0 : OFF, 1: ON"/1 -> Logical Operator4/2
  "Vehicle envelope control switch 0: VEC OFF, 1:VEC ON"/1 -> Logical Operator3/2
  "Tire envelope control switch 0: TEC OFF , 1: TEC ON"/1 -> Logical Operator2/2
  Logical Operator4/1 -> [df_sw]
  Logical Operator2/1 -> [TEC_sw]
  Logical Operator3/1 -> [VEC_sw]
  "drive switch 0 : OFF(no driving force), 1 : ON"/1 -> [D_sw]
  Manual Switch/1 -> [sliplimit_sw]
  Step/1 -> Manual Switch/2
  "Slip limit control switch 0: OFF , 1: ON"/1 -> Manual Switch/1
  "Safe area 0 : small, 1: large"/1 -> [Boundary_sw]
  Diff_sw (VEC_sw)/1 -> [Diff_sw], Logical Operator1/1
  Gain_sw/1 -> Logical Operator1/2
  Triggered Subsystem1/1(Out1) -> Unit Delay/1
  Unit Delay/1 -> Triggered Subsystem1/1(In1), [Diff_gain]
  Logical Operator1/1 -> Delay/1(In1), Logical Operator5/1
  Delay/1(Out1) -> Logical Operator5/2
  Logical Operator5/1 -> Triggered Subsystem1/Trigger

== system debugECDD/Envelope control with Differential drive/envelope controller with DD/Estimator switch ==
  "Beta estimation switch 0: from estimator, 1:from GPS" : Constant  OutDataType=sfix(16)  OutScaling=2^0
  "Vx switch 0: from wheel speed, 1:from GPS" : Constant  OutDataType=sfix(16)  OutScaling=2^0
  "lateral weight shift switch 0: OFF, 1:ON" : Constant  OutDataType=sfix(16)  OutScaling=2^0
  "longitudinal weight shift swich 0: OFF, 1:ON" : Constant  OutDataType=sfix(16)  OutScaling=2^0
  "muFz estimation switch 0: from estimator, 1:from GPS " : Constant  OutDataType=sfix(16)  OutScaling=2^0
  tag scope: Vx_sw=global, ax_sw=global, ay_sw=global, beta_est_sw=global, muFz_est_sw=global
  wires:
  "lateral weight shift switch 0: OFF, 1:ON"/1 -> [ay_sw]
  "longitudinal weight shift swich 0: OFF, 1:ON"/1 -> [ax_sw]
  "muFz estimation switch 0: from estimator, 1:from GPS "/1 -> [muFz_est_sw]
  "Beta estimation switch 0: from estimator, 1:from GPS"/1 -> [beta_est_sw]
  "Vx switch 0: from wheel speed, 1:from GPS"/1 -> [Vx_sw]

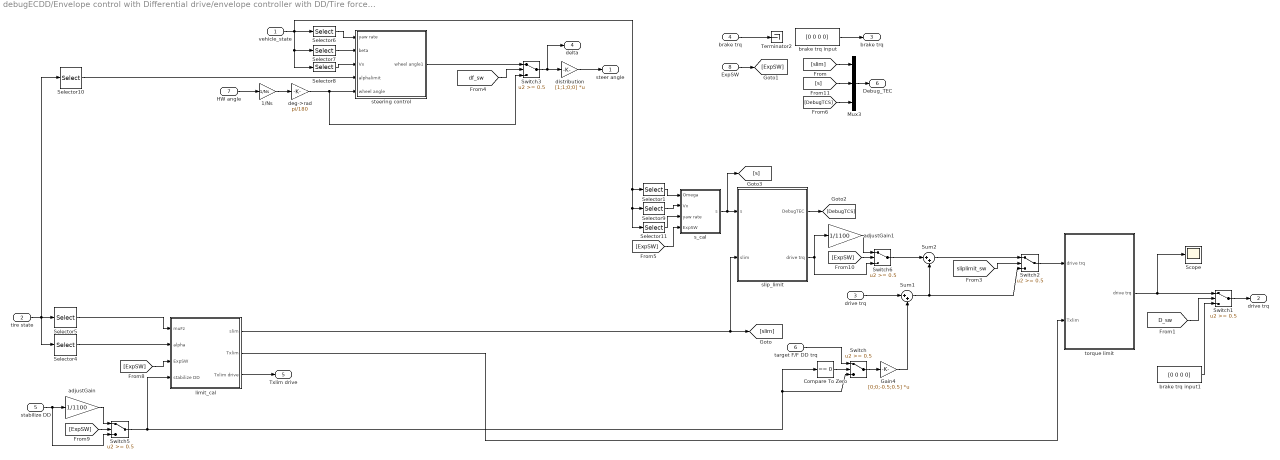
== system debugECDD/Envelope control with Differential drive/envelope controller with DD/Tire force control ==
  vehicle_state : Inport  OutDataType=sfix(16)  OutScaling=2^0
  tire state : Inport  Port=2  OutDataType=sfix(16)  OutScaling=2^0
  "drive trq " : Inport  Port=3  OutDataType=sfix(16)  OutScaling=2^0
  "brake trq " : Inport  Port=4  OutDataType=sfix(16)  OutScaling=2^0
  stabilize DD : Inport  Port=5  OutDataType=sfix(16)  OutScaling=2^0
  target F/F DD trq : Inport  Port=6  OutDataType=sfix(16)  OutScaling=2^0
  HW angle : Inport  Port=7  OutDataType=sfix(16)  OutScaling=2^0
  ExpSW : Inport  Port=8  OutDataType=sfix(16)  OutScaling=2^0
  1/Ns : Gain  Gain=1/Ns  ParameterDataType=sfix(16)  ParameterScaling=2^0  OutDataType=sfix(16)  OutScaling=2^0
  Compare To Zero : simulink/Logic and Bit Operations/Compare To Zero  SystemSampleTime=-1  relop===  LogicOutDataTypeMode=uint8  ZeroCross=off
  Gain4 : Gain  Gain=[0;0;-0.5;0.5]  Multiplication=Matrix(K*u)  ParameterDataType=sfix(16)  ParameterScaling=2^0  OutDataType=sfix(16)  OutScaling=2^0
  Mux3 : Mux  Inputs=3
  Scope : Scope
      settings: YMin=-200  YMax=225  SaveName=ScopeData8
  Selector1 : Selector  InputPortWidth=12  IndexOptions=Index vector (dialog)  Indices=[1:4]  OutputSizes=1
  Selector10 : Selector  InputPortWidth=9  IndexOptions=Index vector (dialog)  Indices=[7:8]  OutputSizes=1
  Selector11 : Selector  InputPortWidth=12  IndexOptions=Index vector (dialog)  Indices=7  OutputSizes=1
  Selector4 : Selector  InputPortWidth=9  IndexOptions=Index vector (dialog)  Indices=[1:2]  OutputSizes=1
  Selector5 : Selector  InputPortWidth=9  IndexOptions=Index vector (dialog)  Indices=[3:6]  OutputSizes=1
  Selector6 : Selector  InputPortWidth=12  IndexOptions=Index vector (dialog)  Indices=7  OutputSizes=1
  Selector7 : Selector  InputPortWidth=12  IndexOptions=Index vector (dialog)  Indices=12  OutputSizes=1
  Selector8 : Selector  InputPortWidth=12  IndexOptions=Index vector (dialog)  Indices=5  OutputSizes=1
  Selector9 : Selector  InputPortWidth=12  IndexOptions=Index vector (dialog)  Indices=5  OutputSizes=1
  Sum1 : Sum  Inputs=|++  OutDataType=sfix(16)  OutScaling=2^0
  Sum2 : Sum  Inputs=|++  OutDataType=sfix(16)  OutScaling=2^0
  Switch : Switch  Threshold=0.5  OutDataType=sfix(16)  OutScaling=2^0
  Switch{1..3,5..6} (5 alike) : Switch  Threshold=0.5
  Terminator2 : Terminator
  adjustGain : Gain  Gain=1/1100  ParameterDataType=sfix(16)  ParameterScaling=2^0  OutDataType=sfix(16)  OutScaling=2^0
  adjustGain1 : Gain  Gain=1/1100  ParameterDataType=sfix(16)  ParameterScaling=2^0  OutDataType=sfix(16)  OutScaling=2^0
  brake trq input : Constant  Value=[0 0 0 0]  OutDataType=sfix(16)  OutScaling=2^0
  brake trq input1 : Constant  Value=[0 0 0 0]  OutDataType=sfix(16)  OutScaling=2^0
  deg->rad : Gain  Gain=pi/180  ParameterDataType=sfix(16)  ParameterScaling=2^0  OutDataType=sfix(16)  OutScaling=2^0
  distribution : Gain  Gain=[1;1;0;0]  Multiplication=Matrix(K*u)  ParameterDataType=sfix(16)  ParameterScaling=2^0  OutDataType=sfix(16)  OutScaling=2^0
  limit_cal : Subsystem
  "s_cal " : Subsystem
  slip_limit : Subsystem
  steering control : Subsystem
  torque limit : Subsystem
  steer angle : Outport  OutDataType=sfix(16)  OutScaling=2^0
  drive trq : Outport  Port=2  OutDataType=sfix(16)  OutScaling=2^0
  brake trq : Outport  Port=3  OutDataType=sfix(16)  OutScaling=2^0
  delta : Outport  Port=4  OutDataType=sfix(16)  OutScaling=2^0
  Txlim drive : Outport  Port=5  OutDataType=sfix(16)  OutScaling=2^0
  Debug_TEC : Outport  Port=6  OutDataType=sfix(16)  OutScaling=2^0
  wires:
  [s] -> Mux3/2
  [DebugTCS] -> Mux3/3
  slip_limit/2(drive trq) -> Switch6/3, adjustGain1/1
  adjustGain1/1 -> Switch6/1
  [ExpSW] -> Switch6/2
  adjustGain/1 -> Switch5/1
  stabilize DD/1 -> adjustGain/1, Switch5/3
  [ExpSW] -> Switch5/2
  [ExpSW] -> limit_cal/3(ExpSW)
  ExpSW/1 -> [ExpSW]
  [ExpSW] -> "s_cal "/4(ExpSW)
  Selector11/1 -> "s_cal "/3(yaw rate)
  Mux3/1 -> Debug_TEC/1
  [slim] -> Mux3/1
  slip_limit/1(DebugTEC) -> [DebugTCS]
  Selector10/1 -> steering control/4(alphalimit)
  Selector9/1 -> "s_cal "/2(Vx)
  torque limit/1(drive trq) -> Scope/1, Switch1/1
  Selector7/1 -> steering control/2(beta)
  Selector6/1 -> steering control/1(yaw rate)
  vehicle_state/1 -> Selector8/1, Selector7/1, Selector11/1, Selector9/1, Selector1/1, Selector6/1
  Selector5/1 -> limit_cal/1(muFz)
  Selector4/1 -> limit_cal/2(alpha)
  Selector8/1 -> steering control/3(Vx)
  deg->rad/1 -> Switch3/3, steering control/5(wheel angle)
  1/Ns/1 -> deg->rad/1
  distribution/1 -> steer angle/1
  HW angle/1 -> 1/Ns/1
  steering control/1(wheel angle1) -> Switch3/1
  Switch3/1 -> delta/1, distribution/1
  [df_sw] -> Switch3/2
  limit_cal/2(Txlim) -> torque limit/2(Txlim)
  tire state/1 -> Selector10/1, Selector4/1, Selector5/1
  brake trq input/1 -> brake trq/1
  "brake trq "/1 -> Terminator2/1
  Selector1/1 -> "s_cal "/1(Omega)
  "s_cal "/1(s) -> slip_limit/1(s), [s]
  Switch1/1 -> drive trq/1
  brake trq input1/1 -> Switch1/3
  [D_sw] -> Switch1/2
  [sliplimit_sw] -> Switch2/2
  limit_cal/3(Txlim drive) -> Txlim drive/1
  Switch/1 -> Gain4/1
  Switch6/1 -> Sum2/1
  Sum2/1 -> Switch2/1
  Sum1/1 -> Sum2/2, Switch2/3
  Switch2/1 -> torque limit/1("drive trq ")
  limit_cal/1(slim) -> slip_limit/2(slim), [slim]
  Switch5/1 -> limit_cal/4(stabilize DD), Compare To Zero/1, Switch/3
  "drive trq "/1 -> Sum1/1
  Compare To Zero/1 -> Switch/2
  Gain4/1 -> Sum1/2
  target F/F DD trq/1 -> Switch/1

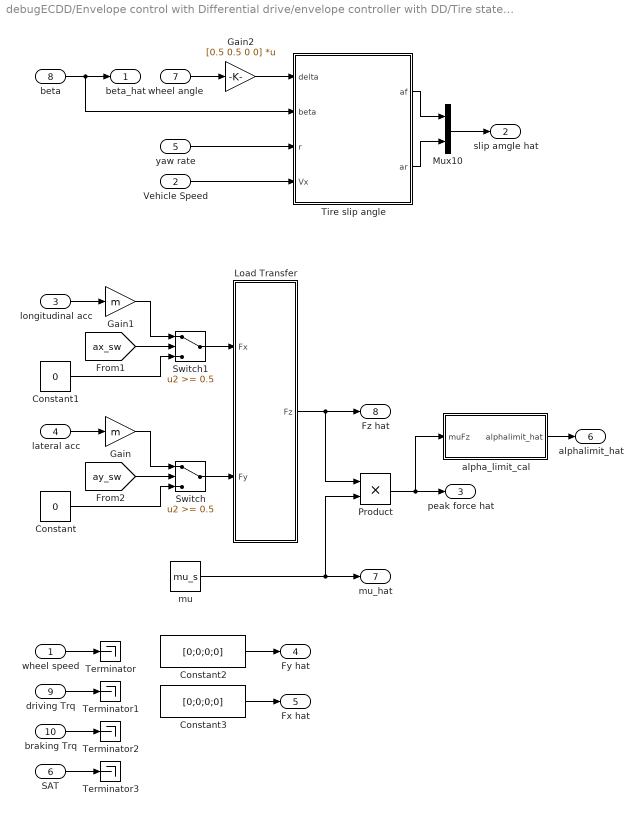
== system debugECDD/Envelope control with Differential drive/envelope controller with DD/Tire state estimation ==
  wheel speed : Inport  OutDataType=sfix(16)  OutScaling=2^0
  Vehicle Speed : Inport  Port=2  OutDataType=sfix(16)  OutScaling=2^0
  longitudinal acc : Inport  Port=3  OutDataType=sfix(16)  OutScaling=2^0
  lateral acc : Inport  Port=4  OutDataType=sfix(16)  OutScaling=2^0
  yaw rate : Inport  Port=5  OutDataType=sfix(16)  OutScaling=2^0
  SAT : Inport  Port=6  OutDataType=sfix(16)  OutScaling=2^0
  wheel angle : Inport  Port=7  OutDataType=sfix(16)  OutScaling=2^0
  beta : Inport  Port=8  OutDataType=sfix(16)  OutScaling=2^0
  driving Trq : Inport  Port=9  OutDataType=sfix(16)  OutScaling=2^0
  braking Trq : Inport  Port=10  OutDataType=sfix(16)  OutScaling=2^0
  Constant : Constant  Value=0  OutDataType=sfix(16)  OutScaling=2^0
  Constant1 : Constant  Value=0  OutDataType=sfix(16)  OutScaling=2^0
  Constant2 : Constant  Value=[0;0;0;0]  OutDataType=sfix(16)  OutScaling=2^0
  Constant3 : Constant  Value=[0;0;0;0]  OutDataType=sfix(16)  OutScaling=2^0
  Gain : Gain  Gain=m  ParameterDataType=sfix(16)  ParameterScaling=2^0  OutDataType=sfix(16)  OutScaling=2^0
  Gain1 : Gain  Gain=m  ParameterDataType=sfix(16)  ParameterScaling=2^0  OutDataType=sfix(16)  OutScaling=2^0
  Gain2 : Gain  Gain=[0.5 0.5 0 0]  Multiplication=Matrix(K*u)  ParameterDataType=sfix(16)  ParameterScaling=2^0  OutDataType=sfix(16)  OutScaling=2^0
  Load Transfer : Subsystem
  Mux10 : Mux  Inputs=2
  Product : Product  OutDataType=sfix(16)  OutScaling=2^0  RndMeth=Zero
  Switch : Switch  Threshold=0.5  OutDataType=sfix(16)  OutScaling=2^0
  Switch1 : Switch  Threshold=0.5  OutDataType=sfix(16)  OutScaling=2^0
  Terminator{,1..3} (4 alike) : Terminator
  Tire slip angle : Subsystem
  alpha_limit_cal : Subsystem
  mu : Constant  Value=mu_s  OutDataType=sfix(16)  OutScaling=2^0
  beta_hat : Outport  OutDataType=sfix(16)  OutScaling=2^0
  slip amgle hat : Outport  Port=2  OutDataType=sfix(16)  OutScaling=2^0
  peak force hat : Outport  Port=3  OutDataType=sfix(16)  OutScaling=2^0
  Fy hat : Outport  Port=4  OutDataType=sfix(16)  OutScaling=2^0
  Fx hat : Outport  Port=5  OutDataType=sfix(16)  OutScaling=2^0
  alphalimit_hat : Outport  Port=6  OutDataType=sfix(16)  OutScaling=2^0
  mu_hat : Outport  Port=7  OutDataType=sfix(16)  OutScaling=2^0
  Fz hat : Outport  Port=8  OutDataType=sfix(16)  OutScaling=2^0
  wires:
  Constant3/1 -> Fx hat/1
  Constant2/1 -> Fy hat/1
  SAT/1 -> Terminator3/1
  braking Trq/1 -> Terminator2/1
  driving Trq/1 -> Terminator1/1
  wheel speed/1 -> Terminator/1
  Mux10/1 -> slip amgle hat/1
  Tire slip angle/2(ar) -> Mux10/2
  Tire slip angle/1(af) -> Mux10/1
  Vehicle Speed/1 -> Tire slip angle/4(Vx)
  yaw rate/1 -> Tire slip angle/3(r)
  Gain2/1 -> Tire slip angle/1(delta)
  wheel angle/1 -> Gain2/1
  beta/1 -> Tire slip angle/2(beta), beta_hat/1
  Product/1 -> alpha_limit_cal/1(muFz), peak force hat/1
  mu/1 -> Product/2, mu_hat/1
  Switch1/1 -> Load Transfer/1(Fx)
  Gain1/1 -> Switch1/1
  Constant1/1 -> Switch1/3
  [ax_sw] -> Switch1/2
  longitudinal acc/1 -> Gain1/1
  Gain/1 -> Switch/1
  Constant/1 -> Switch/3
  [ay_sw] -> Switch/2
  Switch/1 -> Load Transfer/2(Fy)
  alpha_limit_cal/1(alphalimit_hat) -> alphalimit_hat/1
  Load Transfer/1(Fz) -> Product/1, Fz hat/1
  lateral acc/1 -> Gain/1

== system debugECDD/Envelope control with Differential drive/envelope controller with DD/VSP_cal ==
  wheel speed : Inport  OutDataType=sfix(16)  OutScaling=2^0
  Vehicle Speed : Inport  Port=2  OutDataType=sfix(16)  OutScaling=2^0
  Gain1 : Gain  Gain=[rfl rfr 0 0]/2  Multiplication=Matrix(K*u)  ParameterDataType=sfix(16)  ParameterScaling=2^0  OutDataType=sfix(16)  OutScaling=2^0
  Switch1 : Switch  Threshold=0.5
  Zero-Order Hold1 : ZeroOrderHold  SampleTime=0.002
  prevent zero : Subsystem
  VSP : Outport  OutDataType=sfix(16)  OutScaling=2^0
  wires:
  prevent zero/1(Out1) -> VSP/1
  wheel speed/1 -> Gain1/1
  Vehicle Speed/1 -> Zero-Order Hold1/1
  Zero-Order Hold1/1 -> Switch1/1
  Switch1/1 -> prevent zero/1(In1)
  Gain1/1 -> Switch1/3
  [Vx_sw] -> Switch1/2

== system debugECDD/Envelope control with Differential drive/envelope controller with DD/brake_dynamics ==
  In1 : Inport  OutDataType=sfix(16)  OutScaling=2^0
  Demux : Demux
  Discrete Transfer Fcn{,1..3} (4 alike) : DiscreteTransferFcn  Numerator=0.3297  Denominator=[1 -0.6703]  SampleTime=0.002
  Mux : Mux
  Out1 : Outport  OutDataType=sfix(16)  OutScaling=2^0
  wires:
  Discrete Transfer Fcn3/1 -> Mux/4
  Discrete Transfer Fcn2/1 -> Mux/3
  Discrete Transfer Fcn1/1 -> Mux/2
  Discrete Transfer Fcn/1 -> Mux/1
  Demux/4 -> Discrete Transfer Fcn3/1
  Demux/3 -> Discrete Transfer Fcn2/1
  Demux/2 -> Discrete Transfer Fcn1/1
  Demux/1 -> Discrete Transfer Fcn/1
  Mux/1 -> Out1/1
  In1/1 -> Demux/1
